simulink model "OCTModel_for_lin"  (R2020a)
settings: Solver=ode23s  StartTime=0.0  StopTime=simParams.duration.Value  FixedStep=0.1  MaxStep=0.1*sqrt(simParams.lengthScaleFactor.Value)  RelTol=1e-3  AbsTol=1e-3
undefined symbols (not defined in the file): dragTurbineManta, dragTurbineManta_ul, env, initializeBussesFromBlock, initializeVariantsFromBlock, plant, PLANT, plant_cl, plantManta2Rot, plantManta2Rot_cl, sixDoFDynamics, sixDoFDynamics_cl, sixDoFDynamicsCoupledFossen, tether000, tether000_cl, tethers, tethers_cl, thr, twoNodeTether, twoNodeTether_cl, vehicle, VEHICLE, vehicle_cl, vehicleManta2Rot, vehicleManta2Rot_cl, vhcl
libraries: vrlib x11, environment_cl x1, flightController_cl x1, gndStnController_cl x1, hiLvlController_cl x1, plantDOE_cl x1, plantManta_cl x1, dspstat3 x1, groundStation_cl x1, NNodeTether_cl x1, nodeDragForce_ul x1, nodeNetBuoyForce_ul x1
PreSaveFcn:
  | % Callback to reset the view so that the
  | % the next person to open isn't totally lost.
  | hilite_system('OCTModel_for_lin/plant');
  | hilite_system('OCTModel_for_lin/plant','none');
  | set_param(gcs,'Zoomfactor','fit to view')
settings Model: ExtModeTrigDuration=100  Creator=mcobb  LastModifiedBy=andre
settings SolverCC: AlgebraicLoopSolver=LineSearch  SolverResetMethod=Robust
settings DataIOCC: ExternalInput=getinputstruct(op_trim1)  InitialState=getstatestruct(op_trim1)  SaveFinalState=on  SaveOutput=off  SaveState=on  DSMLogging=off  ReturnWorkspaceOutputs=off  StateSaveName=tmp_raccel_xout
settings OptimizationCC: EfficientMapNaN2IntZero=off
settings DebuggingCC: SignalRangeChecking=error  AlgebraicLoopMsg=none  ArtificialAlgebraicLoopMsg=none  ArithmeticOperatorsInVariantConditions=warning
settings HardwareCC: TargetBitPerPointer=64  TargetBitPerSizeT=64  TargetBitPerPtrDiffT=64  TargetLongLongMode=on  TargetIntDivRoundTo=Zero  TargetEndianess=LittleEndian  TargetWordSize=64  TargetHWDeviceType=MATLAB Host  ProdEqTarget=off
settings SFSimCC: CustomCodeUndefinedFunction=UseInterfaceOnly
settings CodeAppCC: MaxIdLength=128
settings GRTTargetCC: TargetLangStandard=C89/C90 (ANSI)  CombineOutputUpdateFcns=off  GRTInterface=on

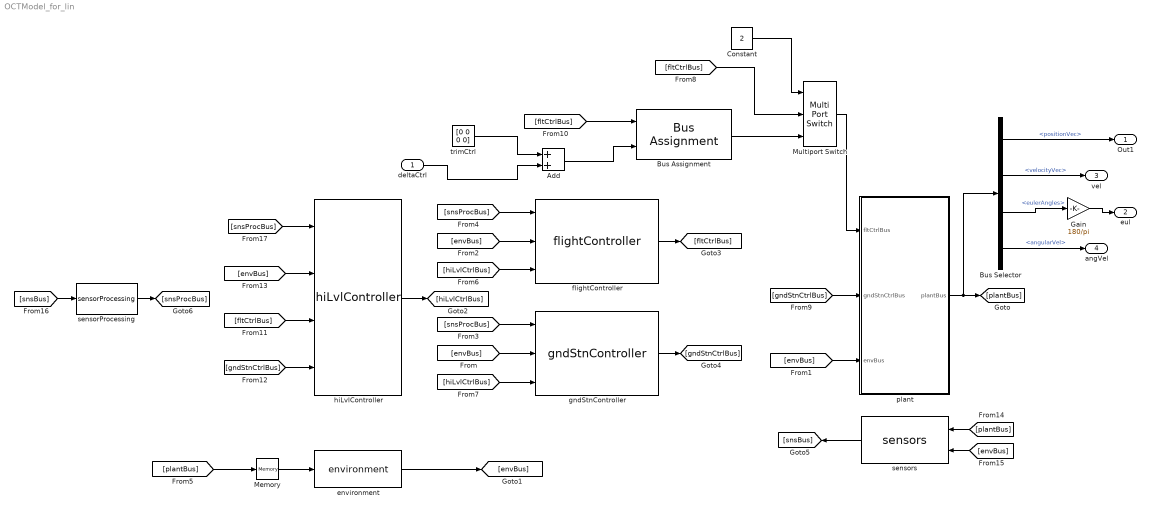
== system OCTModel_for_lin ==
  deltaCtrl : Inport  PortDimensions=4
  Add : Sum
  Bus Assignment : BusAssignment  AssignedSignals=ctrlSurfDeflection
  Bus Selector : BusSelector  OutputSignals=positionVec,velocityVec,eulerAngles,angularVel
  Constant : Constant  Value=2
  Gain : Gain  Gain=180/pi
  Memory : Memory
  Multiport Switch : MultiPortSwitch  Inputs=2
  environment : environment_cl/environment  SystemSampleTime=-1  Latency=0  AutoFrameSizeCalculation=off
  flightController : flightController_cl/flightController  SystemSampleTime=-1  Latency=0  AutoFrameSizeCalculation=off
  gndStnController : gndStnController_cl/gndStnController  SystemSampleTime=-1  Latency=0  AutoFrameSizeCalculation=off
  hiLvlController : hiLvlController_cl/hiLvlController  SystemSampleTime=-1  Latency=0  AutoFrameSizeCalculation=off
  plant : Subsystem  AncestorBlock=plant_cl/plant  Variant=on
  sensorProcessing : sensorProcessing_cl/sensorProcessing  SystemSampleTime=-1  Latency=0  AutoFrameSizeCalculation=off
  sensors : sensors_cl/sensors  SystemSampleTime=-1  Latency=0  AutoFrameSizeCalculation=off
  trimCtrl : Constant  Value=[0 0 0 0]
  Out1 : Outport
  eul : Outport  Port=2
  vel : Outport  Port=3
  angVel : Outport  Port=4
  wires:
  Memory/1 -> environment/1
  [envBus] -> gndStnController/2
  [snsProcBus] -> gndStnController/1
  [snsProcBus] -> flightController/1
  [snsProcBus] -> hiLvlController/1
  flightController/1 -> [fltCtrlBus]
  gndStnController/1 -> [gndStnCtrlBus]
  [envBus] -> hiLvlController/2
  [fltCtrlBus] -> hiLvlController/3
  [gndStnCtrlBus] -> hiLvlController/4
  [plantBus] -> Memory/1
  [hiLvlCtrlBus] -> flightController/3
  [hiLvlCtrlBus] -> gndStnController/3
  hiLvlController/1 -> [hiLvlCtrlBus]
  [envBus] -> flightController/2
  [plantBus] -> sensors/1
  [envBus] -> sensors/2
  sensors/1 -> [snsBus]
  [snsBus] -> sensorProcessing/1
  sensorProcessing/1 -> [snsProcBus]
  plant/1(plantBus) -> Bus Selector/1, [plantBus]
  [gndStnCtrlBus] -> plant/2(gndStnCtrlBus)
  [envBus] -> plant/3(envBus)
  Bus Selector/2 -> vel/1  "<velocityVec>"
  Bus Selector/3 -> Gain/1  "<eulerAngles>"
  Bus Selector/4 -> angVel/1  "<angularVel>"
  trimCtrl/1 -> Add/1
  Add/1 -> Bus Assignment/2
  [fltCtrlBus] -> Bus Assignment/1
  [fltCtrlBus] -> Multiport Switch/2
  Multiport Switch/1 -> plant/1(fltCtrlBus)
  Constant/1 -> Multiport Switch/1
  Bus Assignment/1 -> Multiport Switch/3
  environment/1 -> [envBus]
  Bus Selector/1 -> Out1/1  "<positionVec>"
  Gain/1 -> eul/1
  deltaCtrl/1 -> Add/2

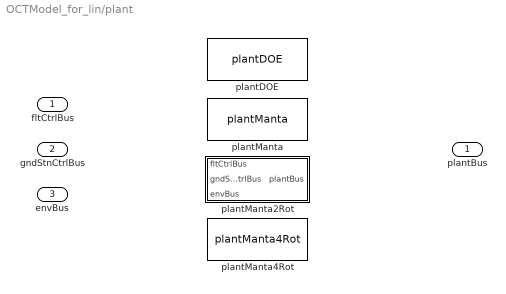
== system OCTModel_for_lin/plant ==
  fltCtrlBus : Inport
  gndStnCtrlBus : Inport  Port=2
  envBus : Inport  Port=3
  plantDOE : plantDOE_cl/plantDOE  SystemSampleTime=-1  VariantControl=strcmpi(PLANT,'plantDOE')  Latency=0  AutoFrameSizeCalculation=off
  plantManta : plantManta_cl/plantManta  SystemSampleTime=-1  VariantControl=strcmpi(PLANT,'plantManta')  Latency=0  AutoFrameSizeCalculation=off
  plantManta2Rot : Subsystem  AncestorBlock=plantManta2Rot_cl/plantManta2Rot  LoadFcn=initializeBussesFromBlock(gcb)  InitFcn=initializeBussesFromBlock(gcb)  StartFcn=initializeBussesFromBlock(gcb)  VariantControl=strcmpi(PLANT,'plantManta2Rot')
  plantManta4Rot : plantManta4Rot_cl/plantManta4Rot  SystemSampleTime=-1  VariantControl=strcmpi(PLANT,'plantManta4Rot')  Latency=0  AutoFrameSizeCalculation=off
  plantBus : Outport

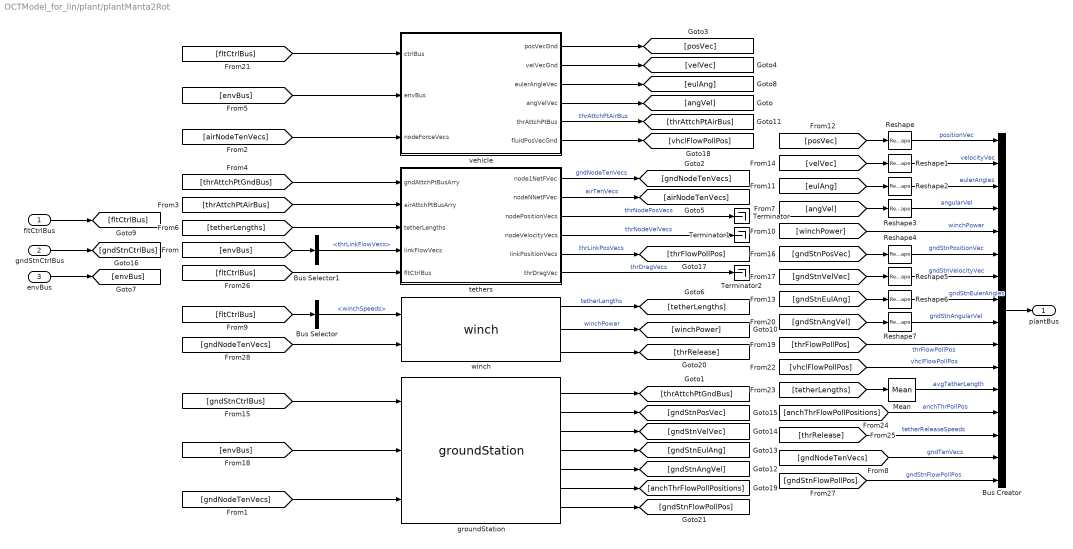
== system OCTModel_for_lin/plant/plantManta2Rot ==
  fltCtrlBus : Inport  OutDataTypeStr=Bus: fltCtrlBus
  gndStnCtrlBus : Inport  Port=2  OutDataTypeStr=Bus: gndStnCtrlBus
  envBus : Inport  Port=3  OutDataTypeStr=Bus: envBus
  Bus Creator : BusCreator  Inputs=16  OutDataTypeStr=Bus: plantBus  NonVirtualBus=on
  Bus Selector : BusSelector  OutputSignals=winchSpeeds
  Bus Selector1 : BusSelector  OutputSignals=thrLinkFlowVecs
  Mean : dspstat3/Mean  run=off  InputProcessing=Columns as channels (frame based)  reset_popup=None  directionMode=Each column  dimension=1  roiEnable=off  roiType=Rectangles  roiPortion=Entire ROI  roiOutput=Individual statistics for each ROI  roiFlag=off  roundingMode=Floor  overflowMode=off  outputDataTypeStr=Inherit: Same as accumulator  outputMin=[]  outputMax=[]  outputLastDataTypeStr=Inherit: Same as accumulator
  Reshape{,1..7} (8 alike) : Reshape  OutputDimensionality=Column vector (2-D)
  Terminator : Terminator
  Terminator1 : Terminator
  Terminator2 : Terminator
  groundStation : groundStation_cl/groundStation  numNodes=2
  tethers : Subsystem  AncestorBlock=tethers_cl/tethers  LoadFcn=initializeVariantsFromBlock(gcb)  InitFcn=initializeVariantsFromBlock(gcb)  StartFcn=initializeVariantsFromBlock(gcb)  Variant=on
      settings: PreSaveFcn=initializeVariantsFromBlock(gcb)
  vehicle : Subsystem  AncestorBlock=vehicle_cl/vehicle  LoadFcn=initializeVariantsFromBlock(gcb)  InitFcn=initializeVariantsFromBlock(gcb)  StartFcn=initializeVariantsFromBlock(gcb)  Variant=on
      settings: PreSaveFcn=initializeVariantsFromBlock(gcb)
  winch : winch_cl/winch  SystemSampleTime=-1  Latency=0  AutoFrameSizeCalculation=off
  plantBus : Outport  OutDataTypeStr=Bus: plantBus  VectorParamsAs1DForOutWhenUnconnected=off
  wires:
  [fltCtrlBus] -> tethers/5(fltCtrlBus)
  tethers/6(thrDragVec) -> Terminator2/1  "thrDragVecs"
  [gndNodeTenVecs] -> winch/2
  tethers/5(linkPositionVecs) -> [thrFlowPollPos]  "thrLinkPosVecs"
  [gndStnFlowPollPos] -> Bus Creator/16  "gndStnFlowPollPos"
  groundStation/7 -> [gndStnFlowPollPos]
  [gndNodeTenVecs] -> Bus Creator/15  "gndTenVecs"
  [thrRelease] -> Bus Creator/14  "tetherReleaseSpeeds"
  [anchThrFlowPollPositions] -> Bus Creator/13  "anchThrPollPos"
  groundStation/6 -> [anchThrFlowPollPositions]
  Mean/1 -> Bus Creator/12  "avgTetherLength"
  [tetherLengths] -> Mean/1
  Bus Selector1/1 -> tethers/4(linkFlowVecs)  "<thrLinkFlowVecs>"
  [vhclFlowPollPos] -> Bus Creator/11  "vhclFlowPollPos"
  vehicle/6(fluidPosVecGnd) -> [vhclFlowPollPos]
  [thrFlowPollPos] -> Bus Creator/10  "thrFlowPollPos"
  tethers/4(nodeVelocityVecs) -> Terminator1/1  "thrNodeVelVecs"
  winch/3 -> [thrRelease]
  Bus Selector/1 -> winch/1  "<winchSpeeds>"
  gndStnCtrlBus/1 -> [gndStnCtrlBus]
  groundStation/5 -> [gndStnAngVel]
  groundStation/4 -> [gndStnEulAng]
  groundStation/3 -> [gndStnVelVec]
  groundStation/2 -> [gndStnPosVec]
  Reshape7/1 -> Bus Creator/9  "gndStnAngularVel"
  Reshape6/1 -> Bus Creator/8  "gndStnEulerAngles"
  Reshape5/1 -> Bus Creator/7  "gndStnVelocityVec"
  Reshape4/1 -> Bus Creator/6  "gndStnPositionVec"
  [gndStnPosVec] -> Reshape4/1
  [gndStnVelVec] -> Reshape5/1
  [gndStnEulAng] -> Reshape6/1
  [gndStnAngVel] -> Reshape7/1
  [winchPower] -> Bus Creator/5  "winchPower"
  winch/2 -> [winchPower]  "winchPower"
  Reshape3/1 -> Bus Creator/4  "angularVel"
  [angVel] -> Reshape3/1
  [fltCtrlBus] -> Bus Selector/1
  [envBus] -> vehicle/2(envBus)
  [fltCtrlBus] -> vehicle/1(ctrlBus)
  [gndStnCtrlBus] -> groundStation/1
  [envBus] -> groundStation/2
  [tetherLengths] -> tethers/3(tetherLengths)
  [thrAttchPtGndBus] -> tethers/1(gndAttchPtBusArry)
  [thrAttchPtAirBus] -> tethers/2(airAttchPtBusArry)
  [airNodeTenVecs] -> vehicle/3(nodeForceVecs)
  [gndNodeTenVecs] -> groundStation/3
  tethers/3(nodePositionVecs) -> Terminator/1  "thrNodePosVecs"
  tethers/2(nodeNNetFVec) -> [airNodeTenVecs]  "airTenVecs"
  tethers/1(node1NetFVec) -> [gndNodeTenVecs]  "gndNodeTenVecs"
  groundStation/1 -> [thrAttchPtGndBus]
  [envBus] -> Bus Selector1/1
  vehicle/4(angVelVec) -> [angVel]
  vehicle/2(velVecGnd) -> [velVec]
  vehicle/5(thrAttchPtBus) -> [thrAttchPtAirBus]  "thrAttchPtAirBus"
  vehicle/1(posVecGnd) -> [posVec]
  vehicle/3(eulerAngleVec) -> [eulAng]
  [eulAng] -> Reshape2/1
  [velVec] -> Reshape1/1
  [posVec] -> Reshape/1
  winch/1 -> [tetherLengths]  "tetherLengths"
  Reshape1/1 -> Bus Creator/2  "velocityVec"
  Reshape2/1 -> Bus Creator/3  "eulerAngles"
  Reshape/1 -> Bus Creator/1  "positionVec"
  Bus Creator/1 -> plantBus/1
  fltCtrlBus/1 -> [fltCtrlBus]
  envBus/1 -> [envBus]

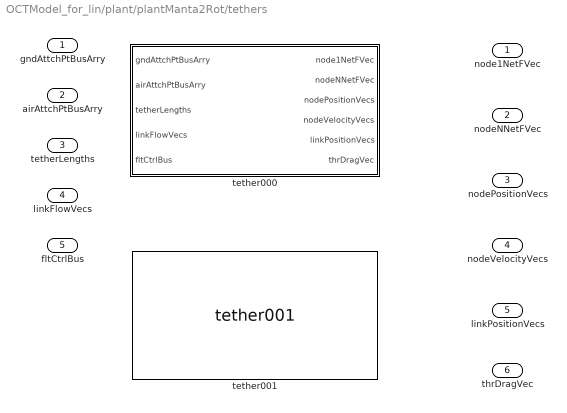
== system OCTModel_for_lin/plant/plantManta2Rot/tethers ==
  gndAttchPtBusArry : Inport
  airAttchPtBusArry : Inport  Port=2
  tetherLengths : Inport  Port=3
  linkFlowVecs : Inport  Port=4
  fltCtrlBus : Inport  Port=5
  tether000 : Subsystem  AncestorBlock=tether000_cl/tether000  Variant=on  VariantControlMode=Label  VariantControl=VSS_tethers_tether000  LabelModeActiveChoice=twoNodeTether  mask{numNodes=thr.numNodes.Value, thrStructure=thr.struct('OCT.tether'), fluidDensity=env.water.density.Value, gravity=env.gravAccel.Value}
      mask prompts: numNodes "Num Nodes"; thrStructure "Tether Structure"; fluidDensity "Fluid Density"; gravity "Gravitational Acceleration"
      mask init:
      | tether000_init
  tether001 : tether001_cl/tether001  VariantControl=VSS_tethers_tether001  thr=thr.tether1  fluidDensity=env.water.density.Value  gravity=env.gravAccel.Value
  node1NetFVec : Outport  VectorParamsAs1DForOutWhenUnconnected=off
  nodeNNetFVec : Outport  Port=2  VectorParamsAs1DForOutWhenUnconnected=off
  nodePositionVecs : Outport  Port=3  VectorParamsAs1DForOutWhenUnconnected=off
  nodeVelocityVecs : Outport  Port=4  VectorParamsAs1DForOutWhenUnconnected=off
  linkPositionVecs : Outport  Port=5  VectorParamsAs1DForOutWhenUnconnected=off
  thrDragVec : Outport  Port=6  VectorParamsAs1DForOutWhenUnconnected=off

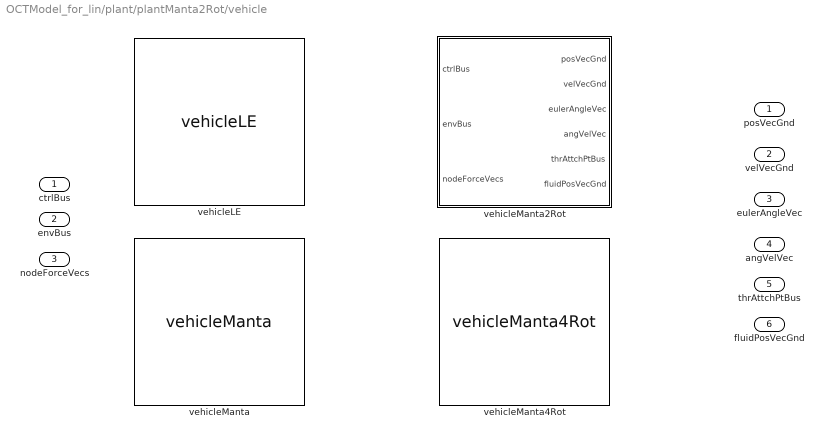
== system OCTModel_for_lin/plant/plantManta2Rot/vehicle ==
  ctrlBus : Inport  OutDataTypeStr=Bus: fltCtrlBus
  envBus : Inport  Port=2  OutDataTypeStr=Bus: envBus
  nodeForceVecs : Inport  Port=3
  vehicleLE : vehicleLE_cl/vehicleLE  VariantControl=strcmpi(VEHICLE,'vehicleLE')  vcl=vhcl  rho=env.water.density.Value  grav=env.gravAccel.Value
  vehicleManta : vehicleManta_cl/vehicleManta  VariantControl=strcmpi(VEHICLE,'vehicleManta')  vcl=vhcl  rho=env.water.density.Value  grav=env.gravAccel.Value
  vehicleManta2Rot : Subsystem  AncestorBlock=vehicleManta2Rot_cl/vehicleManta2Rot  VariantControl=strcmpi(VEHICLE,'vehicleManta2Rot')  mask{vcl=vhcl, rho=env.water.density.Value, grav=env.gravAccel.Value}
      mask prompts: vcl "Vehicle"; rho "Density"; grav "Gravity"
      mask DialogControl Container9 Prompt: General
      mask DialogControl Container5 Prompt: Vehicle object (OCT.vehicle)
      mask DialogControl ParameterGroupVar Prompt: Environment Object (OCT.env)
      mask Display:
      | image('kite2.PNG',[0 0 700 700]/4,'on')
      | 
      | port_label('input',1,'ctrlBus')
      | port_label('input',2,'envBus')
      | port_label('input',3,'nodeForceVecs')
      | 
      | port_label('output',1,'posVecGnd')
      | port_label('output',2,'velVecGnd')
      | port_label('output',3,'eulAng')
      | port_label('output',4,'angVelVec')
      | port_label('output',5,'thrAttchPtBus')
      | port_label('output',6,'fluidPosVecGnd')
  vehicleManta4Rot : vehicleManta4Rot_cl/vehicleManta4Rot  VariantControl=strcmpi(VEHICLE,'vehicleManta4Rot')  vcl=vhcl  rho=env.water.density.Value  grav=env.gravAccel.Value
  posVecGnd : Outport  VectorParamsAs1DForOutWhenUnconnected=off
  velVecGnd : Outport  Port=2  VectorParamsAs1DForOutWhenUnconnected=off
  eulerAngleVec : Outport  Port=3  VectorParamsAs1DForOutWhenUnconnected=off
  angVelVec : Outport  Port=4  VectorParamsAs1DForOutWhenUnconnected=off
  thrAttchPtBus : Outport  Port=5  VectorParamsAs1DForOutWhenUnconnected=off
  fluidPosVecGnd : Outport  Port=6  VectorParamsAs1DForOutWhenUnconnected=off

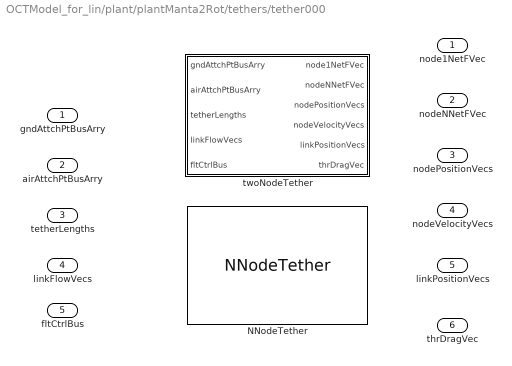
== system OCTModel_for_lin/plant/plantManta2Rot/tethers/tether000 ==
  gndAttchPtBusArry : Inport  OutDataTypeStr=Bus: thrAttachPtKinematicsBus
  airAttchPtBusArry : Inport  Port=2  OutDataTypeStr=Bus: thrAttachPtKinematicsBus
  tetherLengths : Inport  Port=3
  linkFlowVecs : Inport  Port=4
  fltCtrlBus : Inport  Port=5
  NNodeTether : NNodeTether_cl/NNodeTether  VariantControl=NNodeTether  thr=thrStructure  flowDensity=fluidDensity  gravity=gravity
  twoNodeTether : Subsystem  AncestorBlock=twoNodeTether_cl/twoNodeTether  VariantControl=twoNodeTether  mask{thr=thrStructure, flowDensity=fluidDensity, gravity=gravity}
      mask prompts: thr "Tether Structure"; flowDensity "Fluid Density"; gravity "Gravitational Acceleration"
  node1NetFVec : Outport  VectorParamsAs1DForOutWhenUnconnected=off
  nodeNNetFVec : Outport  Port=2  VectorParamsAs1DForOutWhenUnconnected=off
  nodePositionVecs : Outport  Port=3  VectorParamsAs1DForOutWhenUnconnected=off
  nodeVelocityVecs : Outport  Port=4  VectorParamsAs1DForOutWhenUnconnected=off
  linkPositionVecs : Outport  Port=5  VectorParamsAs1DForOutWhenUnconnected=off
  thrDragVec : Outport  Port=6  VectorParamsAs1DForOutWhenUnconnected=off

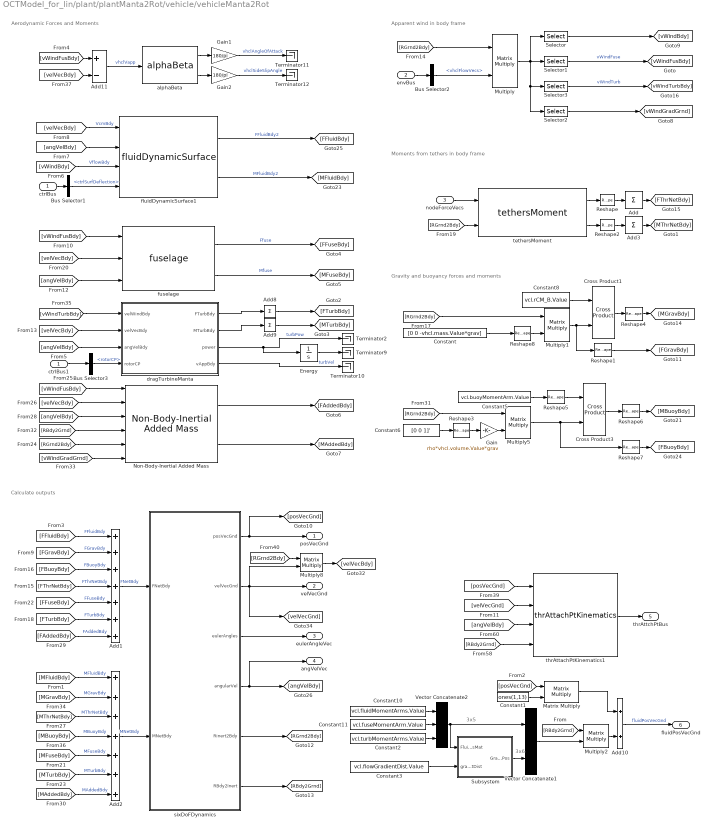
== system OCTModel_for_lin/plant/plantManta2Rot/vehicle/vehicleManta2Rot ==
  note: Aerodynamic Forces and Moments
  note: Moments from tethers in body frame
  note: Gravity and buoyancy forces and moments
  note: Apparent wind in body frame
  note: Calculate outputs
  note: 3x5
  note: 3x6
  ctrlBus : Inport  OutDataTypeStr=Bus: fltCtrlBus
  envBus : Inport  Port=2  OutDataTypeStr=Bus: envBus
  nodeForceVecs : Inport  Port=3
  Add : Sum  Inputs=+  CollapseMode=Specified dimension  CollapseDim=2
  Add1 : Sum  Inputs=+++++++
  Add10 : Sum
  Add11 : Sum  Inputs=+-
  Add2 : Sum  Inputs=+++++++
  Add3 : Sum  Inputs=+  CollapseMode=Specified dimension  CollapseDim=2
  Add8 : Sum  Inputs=1  CollapseMode=Specified dimension  CollapseDim=2
  Add9 : Sum  Inputs=1  CollapseMode=Specified dimension  CollapseDim=2
  Bus Selector1 : BusSelector  OutputSignals=ctrlSurfDeflection
  Bus Selector2 : BusSelector  OutputSignals=vhclFlowVecs
  Bus Selector3 : BusSelector  OutputSignals=rotorCP
  Constant : Constant  Value=[0 0 -vhcl.mass.Value*grav]
  Constant1 : Constant  Value=ones(1,13)  VectorParams1D=off
  Constant10 : Constant  Value=vcl.fluidMomentArms.Value
  Constant11 : Constant  Value=vcl.fuseMomentArm.Value
  Constant2 : Constant  Value=vcl.turbMomentArms.Value
  Constant3 : Constant  Value=vcl.flowGradientDist.Value
  Constant5 : Constant  Value=vcl.buoyMomentArm.Value
  Constant6 : Constant  Value=[0 0 1]'
  Constant8 : Constant  Value=vcl.rCM_B.Value
  Cross Product1 : vrlib/Utilities/Cross Product
  Cross Product3 : vrlib/Utilities/Cross Product
  Energy : Integrator
  Gain : Gain  Gain=rho*vhcl.volume.Value*grav
  Gain1 : Gain  Gain=180/pi
  Gain2 : Gain  Gain=180/pi
  Matrix Multiply : Product  Multiplication=Matrix(*)
  Multiply{,1..2,5,8} (5 alike) : Product  Multiplication=Matrix(*)
  Non-Body-Inertial Added Mass : addedMass_cl/Non-Body-Inertial Added Mass  MaMat=vcl.Ma6x6_LE.Value  rB_LE=vcl.rB_LE.Value  gradDist=vcl.flowGradientDist.Value
  Reshape : Reshape  OutputDimensionality=Customize  OutputDimensions=[3 vcl.numTethers.Value]
  Reshape{1,3..8} (7 alike) : Reshape  OutputDimensionality=Column vector (2-D)
  Reshape2 : Reshape  OutputDimensionality=Customize  OutputDimensions=[3 vcl.numTethers.Value]
  Selector : Selector  NumberOfDimensions=2  InputPortWidth=3  IndexOptions=Select all,Index vector (dialog)  Indices=[1 3],1:4  OutputSizes=1,1
  Selector1 : Selector  NumberOfDimensions=2  InputPortWidth=3  IndexOptions=Select all,Index vector (dialog)  Indices=[1 3],5  OutputSizes=1,1
  Selector2 : Selector  NumberOfDimensions=2  InputPortWidth=3  IndexOptions=Select all,Index vector (dialog)  Indices=[1 3],8:13  OutputSizes=1,1
  Selector3 : Selector  NumberOfDimensions=2  InputPortWidth=3  IndexOptions=Select all,Index vector (dialog)  Indices=[1 3],6:7  OutputSizes=1,1
  Subsystem : Subsystem
  Terminator{2,9..12} (5 alike) : Terminator
  Vector Concatenate1 : Concatenate  Mode=Multidimensional array  ConcatenateDimension=2
  Vector Concatenate2 : Concatenate  NumInputs=3  Mode=Multidimensional array  ConcatenateDimension=2
  alphaBeta : alphaBeta_ul/alphaBeta  SystemSampleTime=-1  Latency=0  AutoFrameSizeCalculation=off
  ctrlBus1 : InportShadow  OutDataTypeStr=Bus: fltCtrlBus
  dragTurbineManta : Subsystem  AncestorBlock=dragTurbineManta_ul/dragTurbineManta  TreatAsAtomicUnit=on  mask{rho_fluid=rho, turb_struct=vcl.struct('OCT.turb')}
      mask prompts: rho_fluid "Fluid density"; turb_struct "Turbines structure"
  fluidDynamicSurface1 : Copy_of_fluidDynamicSurface_cl/fluidDynamicSurface  vcl=vcl  fluidDensity=env.water.density.Value  fluidMomentArms=vcl.fluidMomentArms.Value  fluidRefArea=vcl.fluidRefArea.Value  wingTips=vcl.wingTipPositions.Value
  fuselage : fuselage_cl/fuselage  momArm=vcl.fuseMomentArm.Value  fus=vcl.fuse  fusRhoDa=rho
  sixDoFDynamics : Subsystem  AncestorBlock=sixDoFDynamics_cl/sixDoFDynamics  LoadFcn=initializeVariantsFromBlock(gcb)  InitFcn=initializeVariantsFromBlock(gcb)  Variant=on  mask{vcl=vcl}
      mask prompts: vcl "vehicle object"
  tethersMoment : tethersMoment_cl/tethersMoment  arms=vcl.struct('OCT.thrAttch')
  thrAttachPtKinematics1 : thrAttachPtKinematics_ul/thrAttachPtKinematics  atchPts=vcl.struct('OCT.thrAttch')
  posVecGnd : Outport  VectorParamsAs1DForOutWhenUnconnected=off
  velVecGnd : Outport  Port=2  VectorParamsAs1DForOutWhenUnconnected=off
  eulerAngleVec : Outport  Port=3  VectorParamsAs1DForOutWhenUnconnected=off
  angVelVec : Outport  Port=4  VectorParamsAs1DForOutWhenUnconnected=off
  thrAttchPtBus : Outport  Port=5  VectorParamsAs1DForOutWhenUnconnected=off
  fluidPosVecGnd : Outport  Port=6  VectorParamsAs1DForOutWhenUnconnected=off
  wires:
  [velVecBdy] -> fluidDynamicSurface1/1  "VcmBdy"
  [angVelBdy] -> fluidDynamicSurface1/2
  [vWindBdy] -> fluidDynamicSurface1/3  "VflowBdy"
  Bus Selector1/1 -> fluidDynamicSurface1/4  "<ctrlSurfDeflection>"
  fluidDynamicSurface1/2 -> [MFluidBdy]  "MFluidBdy2"
  fluidDynamicSurface1/1 -> [FFluidBdy]  "FFluidBdy2"
  Gain2/1 -> Terminator12/1  "vhclSideSlipAngle"
  alphaBeta/1 -> Gain1/1
  Gain1/1 -> Terminator11/1  "vhclAngleOfAttack"
  alphaBeta/2 -> Gain2/1
  [velVecBdy] -> Add11/2
  Add11/1 -> alphaBeta/1  "vhclVapp"
  [vWindFusBdy] -> Add11/1
  Non-Body-Inertial Added Mass/2 -> [MAddedBdy]
  Non-Body-Inertial Added Mass/1 -> [FAddedBdy]
  dragTurbineManta/4(vAppBdy) -> Terminator10/1  "turbVel"
  Selector3/1 -> [vWindTurbBdy]  "vWindTurb"
  Constant2/1 -> Vector Concatenate2/3
  ctrlBus1/1 -> Bus Selector3/1
  Bus Selector3/1 -> dragTurbineManta/4(rotorCP)  "<rotorCP>"
  [posVecGnd] -> Matrix Multiply/1
  Constant1/1 -> Matrix Multiply/2
  Add10/1 -> fluidPosVecGnd/1  "fluidPosVecGnd"
  Matrix Multiply/1 -> Add10/1
  Multiply2/1 -> Add10/2
  [RBdy2Grnd] -> Multiply2/1
  Vector Concatenate1/1 -> Multiply2/2
  sixDoFDynamics/4(angularVel) -> angVelVec/1, [angVelBdy]
  Subsystem/1(GradientFlowPos) -> Vector Concatenate1/2
  Constant3/1 -> Subsystem/2(gradientDist)
  Vector Concatenate2/1 -> Subsystem/1(FluidCentPosMat), Vector Concatenate1/1
  Constant11/1 -> Vector Concatenate2/2
  Constant10/1 -> Vector Concatenate2/1
  [RBdy2Grnd] -> thrAttachPtKinematics1/4
  [angVelBdy] -> thrAttachPtKinematics1/3
  [velVecGnd] -> thrAttachPtKinematics1/2
  [posVecGnd] -> thrAttachPtKinematics1/1
  sixDoFDynamics/6(RBdy2Inert) -> [RBdy2Grnd]
  sixDoFDynamics/5(Rinert2Bdy) -> [RGrnd2Bdy]
  Add2/1 -> sixDoFDynamics/2(MNetBdy)  "MNetBdy"
  [MAddedBdy] -> Add2/7  "MAddedBdy"
  [MTurbBdy] -> Add2/6  "MTurbBdy"
  [MFuseBdy] -> Add2/5  "MFuseBdy"
  [MBuoyBdy] -> Add2/4  "MBuoyBdy"
  [MThrNetBdy] -> Add2/3  "MThrNetBdy"
  [MGravBdy] -> Add2/2  "MGravBdy"
  [MFluidBdy] -> Add2/1  "MFluidBdy"
  Add1/1 -> sixDoFDynamics/1(FNetBdy)  "FNetBdy"
  [FAddedBdy] -> Add1/7  "FAddedBdy"
  [FTurbBdy] -> Add1/6  "FTurbBdy"
  [FFuseBdy] -> Add1/5  "FFuseBdy"
  [FThrNetBdy] -> Add1/4  "FThrNetBdy"
  [FBuoyBdy] -> Add1/3  "FBuoyBdy"
  [FGravBdy] -> Add1/2  "FGravBdy"
  [FFluidBdy] -> Add1/1  "FFluidBdy"
  Multiply8/1 -> [velVecBdy]
  [RGrnd2Bdy] -> Multiply8/1
  Selector2/1 -> [vWindGradGrnd]
  Selector1/1 -> [vWindFusBdy]  "vWindFuse"
  Selector/1 -> [vWindBdy]
  Multiply/1 -> Selector1/1, Selector3/1, Selector2/1, Selector/1
  Bus Selector2/1 -> Multiply/2  "<vhclFlowVecs>"
  envBus/1 -> Bus Selector2/1
  [RGrnd2Bdy] -> Multiply/1
  Add3/1 -> [MThrNetBdy]
  Add/1 -> [FThrNetBdy]
  Reshape2/1 -> Add3/1
  Reshape/1 -> Add/1
  tethersMoment/2 -> Reshape2/1
  tethersMoment/1 -> Reshape/1
  nodeForceVecs/1 -> tethersMoment/1
  [RGrnd2Bdy] -> tethersMoment/2
  Reshape4/1 -> [MGravBdy]
  Cross Product1/1 -> Reshape4/1
  Constant8/1 -> Cross Product1/1
  Reshape8/1 -> Multiply1/2
  [RGrnd2Bdy] -> Multiply1/1
  Constant/1 -> Reshape8/1
  fuselage/2 -> [MFuseBdy]  "Mfuse"
  fuselage/1 -> [FFuseBdy]  "Ffuse"
  Multiply1/1 -> Cross Product1/2, Reshape1/1
  Reshape1/1 -> [FGravBdy]
  Reshape7/1 -> [FBuoyBdy]
  Multiply5/1 -> Cross Product3/2, Reshape7/1
  Reshape6/1 -> [MBuoyBdy]
  Cross Product3/1 -> Reshape6/1
  Reshape5/1 -> Cross Product3/1
  Constant5/1 -> Reshape5/1
  Gain/1 -> Multiply5/2
  [RGrnd2Bdy] -> Multiply5/1
  Reshape3/1 -> Gain/1
  Constant6/1 -> Reshape3/1
  [vWindGradGrnd] -> Non-Body-Inertial Added Mass/6
  [RGrnd2Bdy] -> Non-Body-Inertial Added Mass/5
  [RBdy2Grnd] -> Non-Body-Inertial Added Mass/4
  [angVelBdy] -> Non-Body-Inertial Added Mass/3
  [velVecBdy] -> Non-Body-Inertial Added Mass/2
  [vWindFusBdy] -> Non-Body-Inertial Added Mass/1
  dragTurbineManta/3(power) -> Energy/1, Terminator2/1  "turbPow"
  Add9/1 -> [MTurbBdy]
  Add8/1 -> [FTurbBdy]
  dragTurbineManta/2(MTurbBdy) -> Add9/1
  dragTurbineManta/1(FTurbBdy) -> Add8/1
  [angVelBdy] -> dragTurbineManta/3(angVelBdy)
  [velVecBdy] -> dragTurbineManta/2(velVecBdy)
  [vWindTurbBdy] -> dragTurbineManta/1(velWindBdy)
  [angVelBdy] -> fuselage/3
  [velVecBdy] -> fuselage/2
  [vWindFusBdy] -> fuselage/1
  ctrlBus/1 -> Bus Selector1/1
  thrAttachPtKinematics1/1 -> thrAttchPtBus/1
  sixDoFDynamics/2(velVecGnd) -> velVecGnd/1, [velVecGnd], Multiply8/2
  sixDoFDynamics/1(posVecGnd) -> posVecGnd/1, [posVecGnd]
  sixDoFDynamics/3(eulerAngles) -> eulerAngleVec/1
  Energy/1 -> Terminator9/1

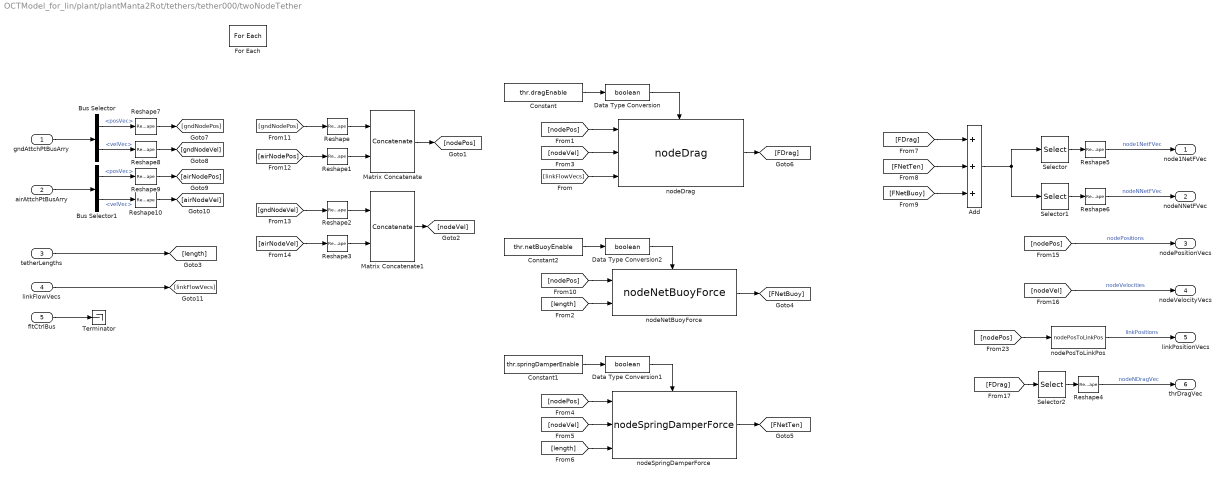
== system OCTModel_for_lin/plant/plantManta2Rot/tethers/tether000/twoNodeTether ==
  gndAttchPtBusArry : Inport  OutDataTypeStr=Bus: thrAttachPtKinematicsBus  Partition=on  PartitionDimension=1  PartitionWidth=1  PartitionOffset=0
  airAttchPtBusArry : Inport  Port=2  OutDataTypeStr=Bus: thrAttachPtKinematicsBus  Partition=on  PartitionDimension=1  PartitionWidth=1  PartitionOffset=0
  tetherLengths : Inport  Port=3  Partition=on  PartitionDimension=1  PartitionWidth=1  PartitionOffset=0
  linkFlowVecs : Inport  Port=4  Partition=on  PartitionDimension=3  PartitionWidth=1  PartitionOffset=0
  fltCtrlBus : Inport  Port=5
  Add : Sum  Inputs=3
  Bus Selector : BusSelector  OutputSignals=posVec,velVec
  Bus Selector1 : BusSelector  OutputSignals=posVec,velVec
  Constant : Constant  Value=thr.dragEnable
  Constant1 : Constant  Value=thr.springDamperEnable
  Constant2 : Constant  Value=thr.netBuoyEnable
  Data Type Conversion : DataTypeConversion  OutDataTypeStr=boolean
  Data Type Conversion1 : DataTypeConversion  OutDataTypeStr=boolean
  Data Type Conversion2 : DataTypeConversion  OutDataTypeStr=boolean
  For Each : ForEach  DisableCoverage=on  IterateSubsysMaskParameter=on,off,off  SubsysMaskParameterIterationDimension=2,1,1
  Matrix Concatenate : Concatenate  Mode=Multidimensional array  ConcatenateDimension=2
  Matrix Concatenate1 : Concatenate  Mode=Multidimensional array  ConcatenateDimension=2
  Reshape{,1..10} (11 alike) : Reshape  OutputDimensionality=Column vector (2-D)
  Selector : Selector  NumberOfDimensions=2  InputPortWidth=3  IndexOptions=Select all,Index vector (dialog)  Indices=[1 3],1  OutputSizes=1,1
  Selector1 : Selector  NumberOfDimensions=2  InputPortWidth=3  IndexOptions=Select all,Index vector (dialog)  Indices=[1 3],2  OutputSizes=1,1
  Selector2 : Selector  NumberOfDimensions=2  InputPortWidth=3  IndexOptions=Select all,Index vector (dialog)  Indices=[1 3],2  OutputSizes=1,1
  Terminator : Terminator
  nodeDrag : nodeDragForce_ul/nodeDrag  flowDensity=flowDensity  thrDiam=thr.diameter  dragCoeff=thr.dragCoeff
  nodeNetBuoyForce : nodeNetBuoyForce_ul/nodeNetBuoyForce  fluidDensity=flowDensity  tetherDensity=thr.density  diameter=thr.diameter  gravity=gravity
  nodePosToLinkPos : nodePosToLinkPos_ul/nodePosToLinkPos  SystemSampleTime=-1  Latency=0  AutoFrameSizeCalculation=off
  nodeSpringDamperForce : nodeSpringDamperForce_ul/nodeSpringDamperForce  mass=thr.vehicleMass  zeta=thr.dampingRatio  diameter=thr.diameter  youngsMod=thr.youngsMod
  node1NetFVec : Outport  ConcatenationDimension=3  VectorParamsAs1DForOutWhenUnconnected=off
  nodeNNetFVec : Outport  Port=2  ConcatenationDimension=3  VectorParamsAs1DForOutWhenUnconnected=off
  nodePositionVecs : Outport  Port=3  ConcatenationDimension=3  VectorParamsAs1DForOutWhenUnconnected=off
  nodeVelocityVecs : Outport  Port=4  ConcatenationDimension=3  VectorParamsAs1DForOutWhenUnconnected=off
  linkPositionVecs : Outport  Port=5  ConcatenationDimension=3  VectorParamsAs1DForOutWhenUnconnected=off
  thrDragVec : Outport  Port=6  ConcatenationDimension=3  VectorParamsAs1DForOutWhenUnconnected=off
  wires:
  fltCtrlBus/1 -> Terminator/1
  Reshape4/1 -> thrDragVec/1  "nodeNDragVec"
  Selector2/1 -> Reshape4/1
  [FDrag] -> Selector2/1
  Reshape6/1 -> nodeNNetFVec/1  "nodeNNetFVec"
  Reshape5/1 -> node1NetFVec/1  "node1NetFVec"
  [nodePos] -> nodePositionVecs/1  "nodePositions"
  [nodeVel] -> nodeVelocityVecs/1  "nodeVelocities"
  nodePosToLinkPos/1 -> linkPositionVecs/1  "linkPositions"
  linkFlowVecs/1 -> [linkFlowVecs]
  [nodePos] -> nodePosToLinkPos/1
  Data Type Conversion2/1 -> nodeNetBuoyForce/Enable
  Constant2/1 -> Data Type Conversion2/1
  Constant1/1 -> Data Type Conversion1/1
  Data Type Conversion1/1 -> nodeSpringDamperForce/Enable
  Data Type Conversion/1 -> nodeDrag/Enable
  Constant/1 -> Data Type Conversion/1
  Reshape10/1 -> [airNodeVel]
  Reshape9/1 -> [airNodePos]
  Reshape8/1 -> [gndNodeVel]
  Reshape7/1 -> [gndNodePos]
  Bus Selector1/1 -> Reshape9/1  "<posVec>"
  airAttchPtBusArry/1 -> Bus Selector1/1
  Bus Selector1/2 -> Reshape10/1  "<velVec>"
  Bus Selector/2 -> Reshape8/1  "<velVec>"
  gndAttchPtBusArry/1 -> Bus Selector/1
  Bus Selector/1 -> Reshape7/1  "<posVec>"
  Matrix Concatenate1/1 -> [nodeVel]
  [nodePos] -> nodeNetBuoyForce/1
  Selector1/1 -> Reshape6/1
  Add/1 -> Selector/1, Selector1/1
  Selector/1 -> Reshape5/1
  [FNetBuoy] -> Add/3
  [FDrag] -> Add/1
  [FNetTen] -> Add/2
  nodeDrag/1 -> [FDrag]
  nodeSpringDamperForce/1 -> [FNetTen]
  nodeNetBuoyForce/1 -> [FNetBuoy]
  [length] -> nodeSpringDamperForce/3
  [nodePos] -> nodeSpringDamperForce/1
  [nodeVel] -> nodeSpringDamperForce/2
  [length] -> nodeNetBuoyForce/2
  tetherLengths/1 -> [length]
  [nodePos] -> nodeDrag/1
  Matrix Concatenate/1 -> [nodePos]
  Reshape2/1 -> Matrix Concatenate1/1
  Reshape3/1 -> Matrix Concatenate1/2
  Reshape1/1 -> Matrix Concatenate/2
  Reshape/1 -> Matrix Concatenate/1
  [airNodeVel] -> Reshape3/1
  [airNodePos] -> Reshape1/1
  [gndNodeVel] -> Reshape2/1
  [gndNodePos] -> Reshape/1
  [nodeVel] -> nodeDrag/2
  [linkFlowVecs] -> nodeDrag/3

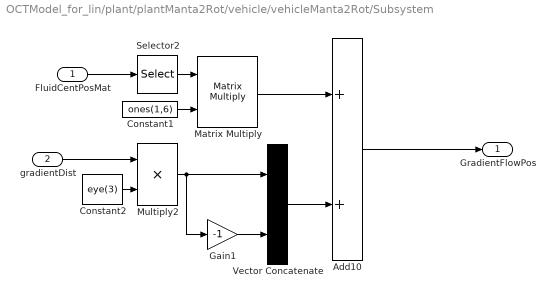
== system OCTModel_for_lin/plant/plantManta2Rot/vehicle/vehicleManta2Rot/Subsystem ==
  FluidCentPosMat : Inport
  gradientDist : Inport  Port=2
  Add10 : Sum
  Constant1 : Constant  Value=ones(1,6)  VectorParams1D=off
  Constant2 : Constant  Value=eye(3)
  Gain1 : Gain  Gain=-1
  Matrix Multiply : Product  Multiplication=Matrix(*)
  Multiply2 : Product
  Selector2 : Selector  NumberOfDimensions=2  InputPortWidth=3  IndexOptions=Select all,Index vector (dialog)  Indices=[1 3],5  OutputSizes=1,1
  Vector Concatenate : Concatenate  Mode=Multidimensional array  ConcatenateDimension=2
  GradientFlowPos : Outport  VectorParamsAs1DForOutWhenUnconnected=off
  wires:
  gradientDist/1 -> Multiply2/1
  Add10/1 -> GradientFlowPos/1
  Constant2/1 -> Multiply2/2
  Gain1/1 -> Vector Concatenate/2
  Matrix Multiply/1 -> Add10/1
  Constant1/1 -> Matrix Multiply/2
  Multiply2/1 -> Vector Concatenate/1, Gain1/1
  Selector2/1 -> Matrix Multiply/1
  Vector Concatenate/1 -> Add10/2
  FluidCentPosMat/1 -> Selector2/1

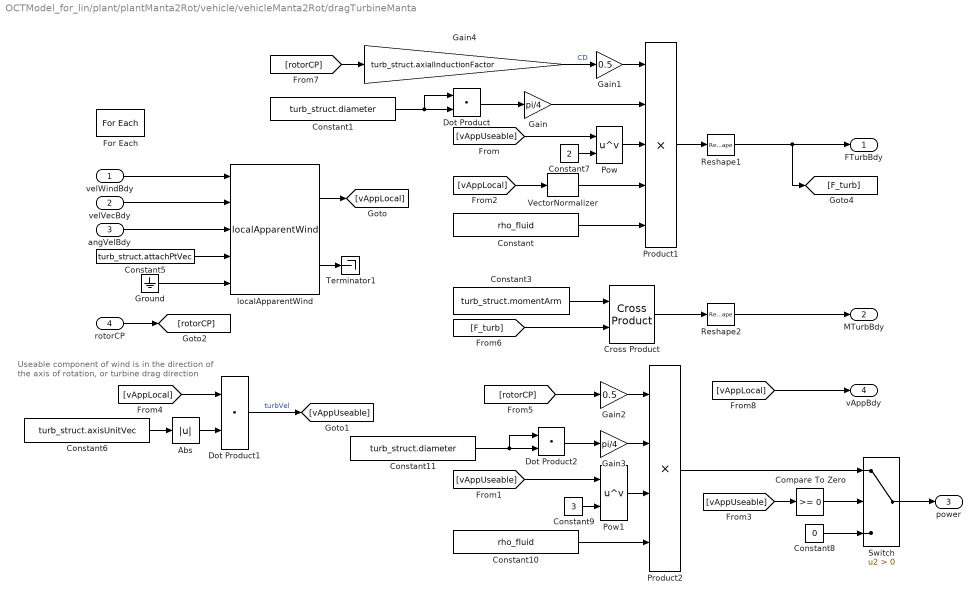
== system OCTModel_for_lin/plant/plantManta2Rot/vehicle/vehicleManta2Rot/dragTurbineManta ==
  note: Useable component of wind is in the direction of
      | the axis of rotation, or turbine drag direction
  velWindBdy : Inport  Partition=on  PartitionDimension=2  PartitionWidth=1  PartitionOffset=0
  velVecBdy : Inport  Port=2
  angVelBdy : Inport  Port=3
  rotorCP : Inport  Port=4
  Abs : Abs
  Compare To Zero : simulink/Logic and Bit Operations/Compare To Zero  relop=>=  OutDataTypeStr=boolean
  Constant : Constant  Value=rho_fluid
  Constant1 : Constant  Value=turb_struct.diameter  VectorParams1D=off
  Constant10 : Constant  Value=rho_fluid
  Constant11 : Constant  Value=turb_struct.diameter  VectorParams1D=off
  Constant3 : Constant  Value=turb_struct.momentArm
  Constant5 : Constant  Value=turb_struct.attachPtVec
  Constant6 : Constant  Value=turb_struct.axisUnitVec
  Constant7 : Constant  Value=2
  Constant8 : Constant  Value=0
  Constant9 : Constant  Value=3
  Cross Product : vrlib/Utilities/Cross Product
  Dot Product : DotProduct  InputSameDT=on  OutDataTypeStr=Inherit: Inherit via internal rule
  Dot Product1 : DotProduct  InputSameDT=on  OutDataTypeStr=Inherit: Inherit via internal rule
  Dot Product2 : DotProduct  InputSameDT=on  OutDataTypeStr=Inherit: Inherit via internal rule
  For Each : ForEach  DisableCoverage=on  IterateSubsysMaskParameter=off,on  SubsysMaskParameterIterationDimension=1,2
  Gain : Gain  Gain=pi/4
  Gain1 : Gain  Gain=0.5
  Gain2 : Gain  Gain=0.5
  Gain3 : Gain  Gain=pi/4
  Gain4 : Gain  Gain=turb_struct.axialInductionFactor
  Ground : Ground
  Pow : Math  Operator=pow  SignedPower=on  RndMeth=Zero  SaturateOnIntegerOverflow=on
  Pow1 : Math  Operator=pow  SignedPower=on  RndMeth=Zero  SaturateOnIntegerOverflow=on
  Product1 : Product  Inputs=5
  Product2 : Product  Inputs=4
  Reshape1 : Reshape  OutputDimensionality=Column vector (2-D)
  Reshape2 : Reshape  OutputDimensionality=Column vector (2-D)
  Switch : Switch  Criteria=u2 > Threshold
  Terminator1 : Terminator
  "VectorNormalizer " : vectorNormalizer_ul/VectorNormalizer   SystemSampleTime=-1  Latency=0  AutoFrameSizeCalculation=off
  localApparentWind : localApparentWind_ul/localApparentWind  SystemSampleTime=-1  Latency=0  AutoFrameSizeCalculation=off
  FTurbBdy : Outport  PortDimensions=[3,1]  ConcatenationDimension=2  VectorParamsAs1DForOutWhenUnconnected=off
  MTurbBdy : Outport  Port=2  PortDimensions=[3,1]  ConcatenationDimension=2  VectorParamsAs1DForOutWhenUnconnected=off
  power : Outport  Port=3  PortDimensions=[1,1]  ConcatenationDimension=2  VectorParamsAs1DForOutWhenUnconnected=off
  vAppBdy : Outport  Port=4  PortDimensions=[3,1]  ConcatenationDimension=2  VectorParamsAs1DForOutWhenUnconnected=off
  wires:
  [vAppLocal] -> vAppBdy/1
  [rotorCP] -> Gain4/1
  [rotorCP] -> Gain2/1
  rotorCP/1 -> [rotorCP]
  [vAppLocal] -> "VectorNormalizer "/1
  Abs/1 -> Dot Product1/2
  localApparentWind/2 -> Terminator1/1
  Ground/1 -> localApparentWind/5
  Cross Product/1 -> Reshape2/1
  Product1/1 -> Reshape1/1
  Product2/1 -> Switch/1
  Gain4/1 -> Gain1/1  "CD"
  Constant3/1 -> Cross Product/1
  [F_turb] -> Cross Product/2
  Reshape1/1 -> FTurbBdy/1, [F_turb]
  Reshape2/1 -> MTurbBdy/1
  velVecBdy/1 -> localApparentWind/2
  angVelBdy/1 -> localApparentWind/3
  velWindBdy/1 -> localApparentWind/1
  localApparentWind/1 -> [vAppLocal]
  Constant5/1 -> localApparentWind/4
  Constant6/1 -> Abs/1
  [vAppUseable] -> Pow/1
  "VectorNormalizer "/1 -> Product1/4
  Constant1/1 -> Dot Product/2, Dot Product/1
  Constant9/1 -> Pow1/2
  Dot Product1/1 -> [vAppUseable]  "turbVel"
  Gain1/1 -> Product1/1
  Constant/1 -> Product1/5
  Constant10/1 -> Product2/4
  Gain2/1 -> Product2/1
  Pow1/1 -> Product2/3
  Pow/1 -> Product1/3
  Constant7/1 -> Pow/2
  Switch/1 -> power/1
  Compare To Zero/1 -> Switch/2
  [vAppUseable] -> Compare To Zero/1
  Constant8/1 -> Switch/3
  [vAppLocal] -> Dot Product1/1
  [vAppUseable] -> Pow1/1
  Dot Product/1 -> Gain/1
  Gain/1 -> Product1/2
  Dot Product2/1 -> Gain3/1
  Constant11/1 -> Dot Product2/2, Dot Product2/1
  Gain3/1 -> Product2/2

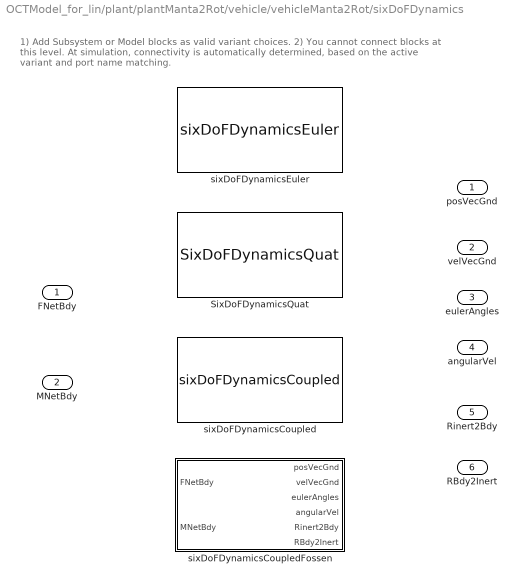
== system OCTModel_for_lin/plant/plantManta2Rot/vehicle/vehicleManta2Rot/sixDoFDynamics ==
  note: 1) Add Subsystem or Model blocks as valid variant choices.
      | 2) You cannot connect blocks at this level. At simulation, connectivity is automatically
      | determined, based on the active variant and port name matching.
  FNetBdy : Inport
  MNetBdy : Inport  Port=2
  SixDoFDynamicsQuat : SixDoFDynamicsQuat_ul/SixDoFDynamicsQuat  VariantControl=VSS_sixDoFDynamics_sixDoFDynamicsQuat  M=vcl.mass.Value  J=vcl.inertia.Value  initPos=vcl.initPosVecGnd.Value  initVel=vcl.initVelVecBdy.Value  initEulAngs=vcl.initEulAng.Value  initAngVel=vcl.initAngVelVec.Value
  sixDoFDynamicsCoupled : sixDoFDynamicsCoupled/sixDoFDynamicsCoupled  VariantControl=VSS_sixDoFDynamics_sixDoFDynamicsCoupled  massMatrix=vcl.M6x6_B.Value  addedMassMatrix=vcl.Ma6x6_LE.Value  rCM_LE=vcl.rCM_LE.Value  initPosCM=vcl.initPosVecGnd.Value  initVelCM=vcl.initVelVecBdy.Value  initEulAngs=vcl.initEulAng.Value  initAngVel=vcl.initAngVelVec.Value
  sixDoFDynamicsCoupledFossen : Subsystem  AncestorBlock=sixDoFDynamicsCoupledFossen/sixDoFDynamicsCoupledFossen  VariantControl=VSS_sixDoFDynamics_sixDoFDynamicsCoupledFossen  mask{MMat=vcl.M6x6_B.Value, MaMat=vcl.Ma6x6_LE.Value, rCM_B=vcl.rCM_B.Value, rB_LE=vcl.rB_LE.Value, initPos=vcl.initPosVecGnd.Value, initVel=vcl.initVelVecBdy.Value, initEulAngs=vcl.initEulAng.Value, initAngVel=vcl.initAngVelVec.Value}
      mask prompts: MMat "6x6 Mass Matrix"; MaMat "6x6 Added Mass Matrix"; rCM_B "Center of mass position vec in body frame"; rB_LE "Body frame origin position vec relative to Leading Edge"; initPos "Initial position"; initVel "Initial velocity"; initEulAngs "Initial Euler Angles"; initAngVel "Initial Angular Velocity Vec"
      mask init:
      | S = @(v) [0 -v(3) v(2);v(3) 0 -v(1);-v(2) v(1) 0];
      | MaAdj = [eye(3) zeros(3);-S(rB_LE) eye(3)]*MaMat;
      | MTot = MMat + MaAdj;
      | MTotInv = inv(MTot);
      | 
      | m = MMat(1,1);
      | J = MMat(4:6,4:6);%About Body Frame
      mask DialogControl Container6 Prompt: Mass Matrices
      mask DialogControl Container4 Prompt: Point Locations
      mask DialogControl Container3 Prompt: Initial Conditions
  sixDoFDynamicsEuler : sixDoFDynamicsEuler_ul/sixDoFDynamicsEuler  VariantControl=VSS_sixDoFDynamics_sixDoFDynamicsEuler  M=vcl.mass.Value  J=vcl.inertia.Value  initPos=vcl.initPosVecGnd.Value  initVel=vcl.initVelVecBdy.Value  initEulAngs=vcl.initEulAng.Value  initAngVel=vcl.initAngVelVec.Value
  posVecGnd : Outport  VectorParamsAs1DForOutWhenUnconnected=off
  velVecGnd : Outport  Port=2  VectorParamsAs1DForOutWhenUnconnected=off
  eulerAngles : Outport  Port=3  VectorParamsAs1DForOutWhenUnconnected=off
  angularVel : Outport  Port=4  VectorParamsAs1DForOutWhenUnconnected=off
  Rinert2Bdy : Outport  Port=5  VectorParamsAs1DForOutWhenUnconnected=off
  RBdy2Inert : Outport  Port=6  VectorParamsAs1DForOutWhenUnconnected=off

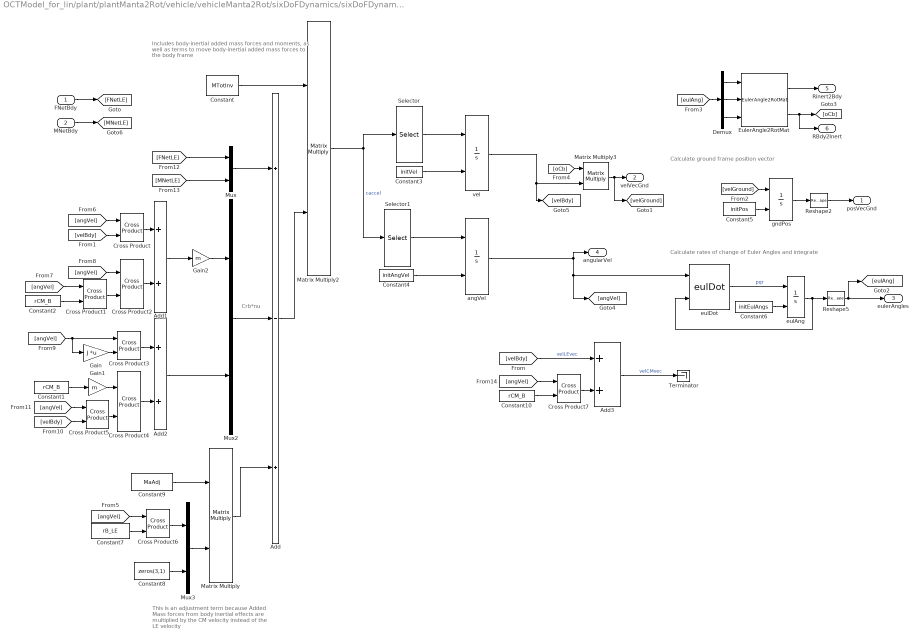
== system OCTModel_for_lin/plant/plantManta2Rot/vehicle/vehicleManta2Rot/sixDoFDynamics/sixDoFDynamicsCoupledFossen ==
  note: Calculate rates of change of Euler Angles and integrate
  note: Calculate ground frame position vector
  note: Includes body-inertial added mass forces and moments,
      | as well as terms to move body-inertial added mass
      | forces to the body frame
  note: This is an adjustment term because Added
      | Mass forces from body inertial effects are
      | multiplied by the CM velocity instead
      | of the LE velocity
  note: Crb*nu
  FNetBdy : Inport
  MNetBdy : Inport  Port=2
  Add : Sum  Inputs=+-+
  Add1 : Sum
  Add2 : Sum
  Add3 : Sum
  Constant : Constant  Value=MTotInv  VectorParams1D=off
  Constant1 : Constant  Value=rCM_B
  Constant10 : Constant  Value=rCM_B
  Constant2 : Constant  Value=rCM_B
  Constant3 : Constant  Value=initVel
  Constant4 : Constant  Value=initAngVel
  Constant5 : Constant  Value=initPos
  Constant6 : Constant  Value=initEulAngs
  Constant7 : Constant  Value=rB_LE
  Constant8 : Constant  Value=zeros(3,1)
  Constant9 : Constant  Value=MaAdj
  Cross Product{,1..7} (8 alike) : vrlib/Utilities/Cross Product
  Demux : Demux  Outputs=3
  EulerAngle2RotMat : eulAng2RotMat_ul/EulerAngle2RotMat  SystemSampleTime=-1  Latency=0  AutoFrameSizeCalculation=off
  Gain : Gain  Gain=J  Multiplication=Matrix(K*u)
  Gain1 : Gain  Gain=m
  Gain2 : Gain  Gain=m
  Matrix Multiply : Product  Multiplication=Matrix(*)
  Matrix Multiply2 : Product  Multiplication=Matrix(*)
  Matrix Multiply3 : Product  Multiplication=Matrix(*)
  Mux : Mux  Inputs=2
  Mux2 : Mux  Inputs=2
  Mux3 : Mux  Inputs=2
  Reshape2 : Reshape  OutputDimensionality=Column vector (2-D)
  Reshape5 : Reshape  OutputDimensionality=Column vector (2-D)
  Selector : Selector  InputPortWidth=6  IndexOptions=Index vector (dialog)  Indices=[1 2 3]  OutputSizes=1
  Selector1 : Selector  InputPortWidth=6  IndexOptions=Index vector (dialog)  Indices=[4 5 6]  OutputSizes=1
  Terminator : Terminator
  angVel : Integrator  InitialConditionSource=external  ContinuousStateAttributes='angVel'
  eulAng : Integrator  InitialConditionSource=external  InitialCondition=initEulAngs  ContinuousStateAttributes='eulAng'
  eulDot : eulDot/eulDot  SystemSampleTime=-1  Latency=0  AutoFrameSizeCalculation=off
  gndPos : Integrator  InitialConditionSource=external  InitialCondition=initPos  ContinuousStateAttributes='gndPos'
  vel : Integrator  InitialConditionSource=external  ContinuousStateAttributes='vel'
  posVecGnd : Outport  VectorParamsAs1DForOutWhenUnconnected=off
  velVecGnd : Outport  Port=2  VectorParamsAs1DForOutWhenUnconnected=off
  eulerAngles : Outport  Port=3  VectorParamsAs1DForOutWhenUnconnected=off
  angularVel : Outport  Port=4  VectorParamsAs1DForOutWhenUnconnected=off
  Rinert2Bdy : Outport  Port=5  VectorParamsAs1DForOutWhenUnconnected=off
  RBdy2Inert : Outport  Port=6  VectorParamsAs1DForOutWhenUnconnected=off
  wires:
  Selector1/1 -> angVel/1
  Selector/1 -> vel/1
  Add3/1 -> Terminator/1  "velCMvec"
  [velBdy] -> Add3/1  "velLEvec"
  Cross Product7/1 -> Add3/2
  [angVel] -> Cross Product7/1
  Constant10/1 -> Cross Product7/2
  [MNetLE] -> Mux/2
  [FNetLE] -> Mux/1
  MNetBdy/1 -> [MNetLE]
  FNetBdy/1 -> [FNetLE]
  Constant9/1 -> Matrix Multiply/1
  Mux3/1 -> Matrix Multiply/2
  Constant8/1 -> Mux3/2
  Cross Product6/1 -> Mux3/1
  Constant7/1 -> Cross Product6/2
  [angVel] -> Cross Product6/1
  Matrix Multiply/1 -> Add/3
  Gain2/1 -> Mux2/1
  Add/1 -> Matrix Multiply2/2
  Add2/1 -> Mux2/2
  Add1/1 -> Gain2/1
  Cross Product4/1 -> Add2/2
  Cross Product3/1 -> Add2/1
  Cross Product5/1 -> Cross Product4/2
  [angVel] -> Cross Product5/1
  [velBdy] -> Cross Product5/2
  Gain1/1 -> Cross Product4/1
  Constant1/1 -> Gain1/1
  Gain/1 -> Cross Product3/2
  [angVel] -> Gain/1, Cross Product3/1
  Cross Product2/1 -> Add1/2
  [angVel] -> Cross Product2/1
  [angVel] -> Cross Product1/1
  Constant2/1 -> Cross Product1/2
  Cross Product1/1 -> Cross Product2/2
  Cross Product/1 -> Add1/1
  [angVel] -> Cross Product/1
  [velBdy] -> Cross Product/2
  Mux2/1 -> Add/2
  Matrix Multiply3/1 -> velVecGnd/1, [velGround]
  [oCb] -> Matrix Multiply3/1
  vel/1 -> Matrix Multiply3/2, [velBdy]
  Constant3/1 -> vel/2
  EulerAngle2RotMat/1 -> Rinert2Bdy/1
  [velGround] -> gndPos/1
  angVel/1 -> angularVel/1, eulDot/1, [angVel]
  Reshape5/1 -> [eulAng], eulerAngles/1
  Constant6/1 -> eulAng/2
  eulAng/1 -> eulDot/2, Reshape5/1
  eulDot/1 -> eulAng/1  "pqr"
  [eulAng] -> Demux/1
  Constant5/1 -> gndPos/2
  Demux/2 -> EulerAngle2RotMat/2
  Reshape2/1 -> posVecGnd/1
  EulerAngle2RotMat/2 -> [oCb], RBdy2Inert/1
  Demux/1 -> EulerAngle2RotMat/1
  Demux/3 -> EulerAngle2RotMat/3
  gndPos/1 -> Reshape2/1
  Constant4/1 -> angVel/2
  Matrix Multiply2/1 -> Selector/1, Selector1/1  "caccel"
  Constant/1 -> Matrix Multiply2/1
  Mux/1 -> Add/1
